simulink model "PHES_Model"  (R2022a)
settings: Solver=VariableStepAuto  StartTime=0.0  StopTime=10.0  RelTol=1e-3
settings Model: Creator=aasav  LastModifiedBy=aasav

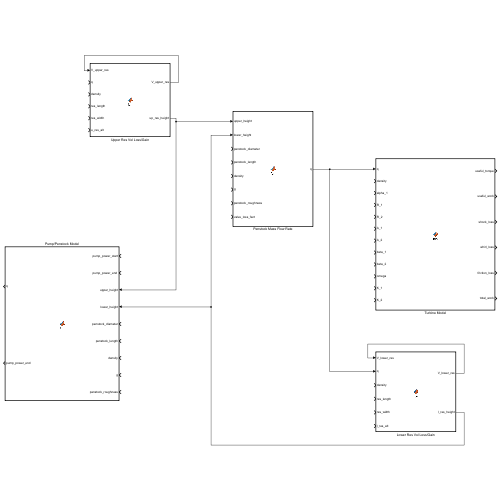
[thumbnail: Simulink's stored preview of the top-level diagram]
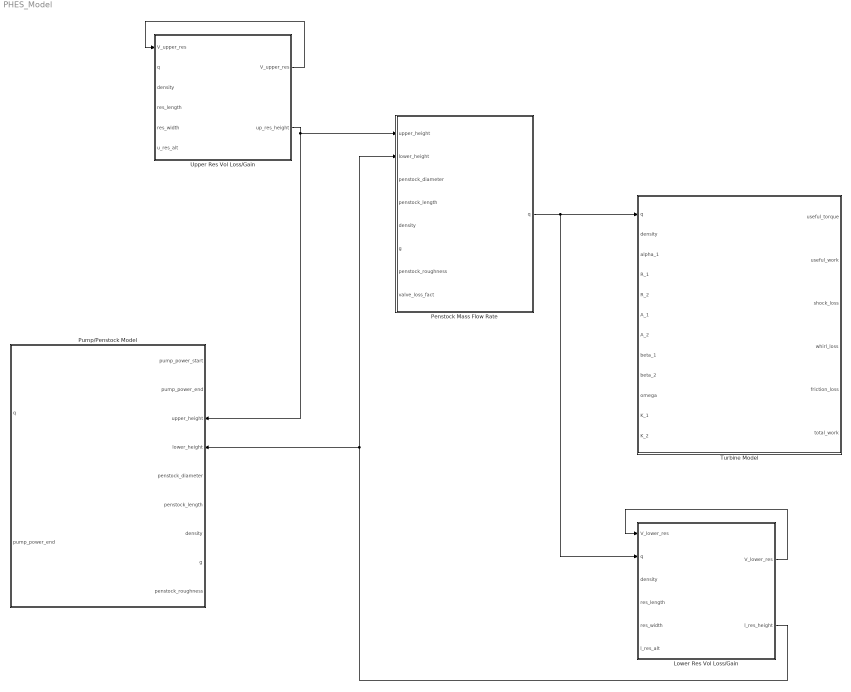
== system PHES_Model ==
  Lower Res Vol Loss/Gain : MATLAB Function  TreatAsAtomicUnit=on
  Penstock Mass Flow Rate : MATLAB Function  TreatAsAtomicUnit=on
  Pump/Penstock Model : MATLAB Function  TreatAsAtomicUnit=on
  Turbine Model : MATLAB Function  TreatAsAtomicUnit=on
  Upper Res Vol Loss/Gain : MATLAB Function  TreatAsAtomicUnit=on
  wires:
  Upper Res Vol Loss/Gain/2(up_res_height) -> Pump/Penstock Model/3(upper_height), Penstock Mass Flow Rate/1(upper_height)
  Penstock Mass Flow Rate/1(q) -> Lower Res Vol Loss/Gain/2(q), Turbine Model/1(q)
  Upper Res Vol Loss/Gain/1(V_upper_res) -> Upper Res Vol Loss/Gain/1("V_upper_res ")
  Lower Res Vol Loss/Gain/2(l_res_height) -> Pump/Penstock Model/4(lower_height), Penstock Mass Flow Rate/2(lower_height)
  Lower Res Vol Loss/Gain/1(V_lower_res) -> Lower Res Vol Loss/Gain/1("V_lower_res ")

== matlab function PHES_Model/Penstock Mass Flow Rate ==
  data: upper_height input; q output; lower_height input; penstock_diameter input; penstock_length input; density input; g input; penstock_roughness input; valve_loss_fact input
function q = fcn(upper_height, lower_height, penstock_diameter, penstock_length, density, g, penstock_roughness, valve_loss_fact)

    q = fcn_penstock_steadystate(upper_height, lower_height, penstock_diameter, penstock_length, density, g, penstock_roughness, valve_loss_fact);

== matlab function PHES_Model/Upper Res Vol Loss//Gain ==
  data: V_upper_res output; V_upper_res input; q input; density input; res_length input; res_width input; up_res_height output; u_res_alt input
function [V_upper_res, up_res_height] = fcn(V_upper_res, q, density, res_length, res_width, u_res_alt)

    [V_upper_res, up_res_height] = fcn_vol_upper(V_upper_res, q, density, res_length, res_width, u_res_alt);

== matlab function PHES_Model/Turbine Model ==
  data: q input; useful_torque output; density input; alpha_1 input; R_1 input; R_2 input; A_1 input; A_2 input; beta_1 input; beta_2 input; omega input; K_1 input; K_2 input; useful_work output; shock_loss output; whirl_loss output; friction_loss output; total_work output
function [useful_torque, useful_work, shock_loss, whirl_loss, friction_loss, total_work] = fcn(q, density, alpha_1, R_1, R_2, A_1, A_2, beta_1, beta_2, omega, K_1, K_2)

    [useful_torque, useful_work, shock_loss, whirl_loss, friction_loss, total_work] = turbine_eqn(q, density, alpha_1, R_1, R_2, A_1, A_2, beta_1, beta_2, omega, K_1, K_2);

== matlab function PHES_Model/Pump//Penstock Model ==
  data: pump_power_start input; q output; pump_power_end input; upper_height input; lower_height input; penstock_diameter input; penstock_length input; density input; g input; penstock_roughness input; pump_power_end output
function [q, pump_power_end] = fcn(pump_power_start, pump_power_end, upper_height, lower_height, penstock_diameter, penstock_length, density, g, penstock_roughness)

    q = fcn_pump_steady_state(pump_power_start, pump_power_end, upper_height, lower_height, penstock_diameter, penstock_length, density, g, penstock_roughness);

== matlab function PHES_Model/Lower Res Vol Loss//Gain ==
  data: V_lower_res input; V_lower_res output; q input; density input; res_length input; res_width input; l_res_height output; l_res_alt input
function [V_lower_res, l_res_height] = fcn(V_lower_res, q, density, res_length, res_width, l_res_alt)

    [V_lower_res, l_res_height] = fcn_vol_lower(V_lower_res, q, density, res_length, res_width, l_res_alt);
